simulink model "Thrust_Direction_quad"  (R2013a)
settings: Solver=ode3  StartTime=0.0  StopTime=10.0  FixedStep=t_s  RelTol=1e-3
libraries: quad_lib x2
settings Model: Creator=diogo  LastModifiedBy=diogo

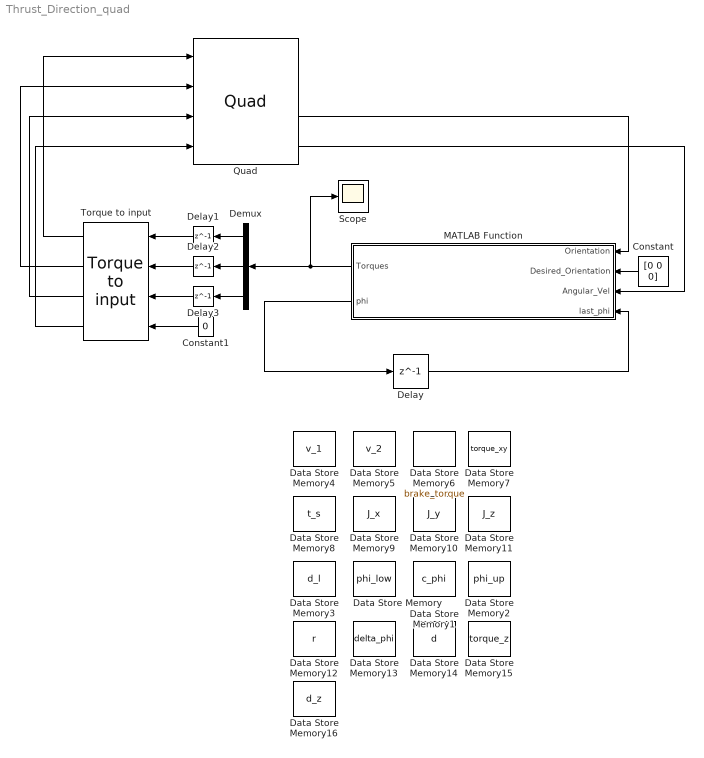
== system Thrust_Direction_quad ==
  Constant : Constant  Value=[0 0 0]
  Constant1 : Constant  Value=0
  Data Store Memory : DataStoreMemory  DataStoreName=phi_low  ReadBeforeWriteMsg=warning  WriteAfterWriteMsg=warning  WriteAfterReadMsg=warning  InitialValue=phi_low  OutDataTypeStr=double
  Data Store Memory1 : DataStoreMemory  DataStoreName=c_phi  ReadBeforeWriteMsg=warning  WriteAfterWriteMsg=warning  WriteAfterReadMsg=warning  InitialValue=c_phi  OutDataTypeStr=double
  Data Store Memory10 : DataStoreMemory  DataStoreName=J_y  ReadBeforeWriteMsg=warning  WriteAfterWriteMsg=warning  WriteAfterReadMsg=warning  InitialValue=J_y  OutDataTypeStr=double
  Data Store Memory11 : DataStoreMemory  DataStoreName=J_z  ReadBeforeWriteMsg=warning  WriteAfterWriteMsg=warning  WriteAfterReadMsg=warning  InitialValue=torque_xy  OutDataTypeStr=double
  Data Store Memory12 : DataStoreMemory  DataStoreName=r  ReadBeforeWriteMsg=warning  WriteAfterWriteMsg=warning  WriteAfterReadMsg=warning  InitialValue=r  OutDataTypeStr=double
  Data Store Memory13 : DataStoreMemory  DataStoreName=delta_phi  ReadBeforeWriteMsg=warning  WriteAfterWriteMsg=warning  WriteAfterReadMsg=warning  InitialValue=delta_phi  OutDataTypeStr=double
  Data Store Memory14 : DataStoreMemory  DataStoreName=d  ReadBeforeWriteMsg=warning  WriteAfterWriteMsg=warning  WriteAfterReadMsg=warning  InitialValue=d  OutDataTypeStr=double
  Data Store Memory15 : DataStoreMemory  DataStoreName=torque_z  ReadBeforeWriteMsg=warning  WriteAfterWriteMsg=warning  WriteAfterReadMsg=warning  InitialValue=torque_z  OutDataTypeStr=double
  Data Store Memory16 : DataStoreMemory  DataStoreName=d_z  ReadBeforeWriteMsg=warning  WriteAfterWriteMsg=warning  WriteAfterReadMsg=warning  InitialValue=d_z  OutDataTypeStr=double
  Data Store Memory2 : DataStoreMemory  DataStoreName=phi_up  ReadBeforeWriteMsg=warning  WriteAfterWriteMsg=warning  WriteAfterReadMsg=warning  InitialValue=phi_up  OutDataTypeStr=double
  Data Store Memory3 : DataStoreMemory  DataStoreName=d_l  ReadBeforeWriteMsg=warning  WriteAfterWriteMsg=warning  WriteAfterReadMsg=warning  InitialValue=d_l  OutDataTypeStr=double
  Data Store Memory4 : DataStoreMemory  DataStoreName=v_1  ReadBeforeWriteMsg=warning  WriteAfterWriteMsg=warning  WriteAfterReadMsg=warning  InitialValue=v_1  OutDataTypeStr=double
  Data Store Memory5 : DataStoreMemory  DataStoreName=v_2  ReadBeforeWriteMsg=warning  WriteAfterWriteMsg=warning  WriteAfterReadMsg=warning  InitialValue=v_2  OutDataTypeStr=double
  Data Store Memory6 : DataStoreMemory  DataStoreName=brake_torque  ReadBeforeWriteMsg=warning  WriteAfterWriteMsg=warning  WriteAfterReadMsg=warning  InitialValue=brake_torque  OutDataTypeStr=double
  Data Store Memory7 : DataStoreMemory  DataStoreName=torque_xy  ReadBeforeWriteMsg=warning  WriteAfterWriteMsg=warning  WriteAfterReadMsg=warning  InitialValue=torque_xy  OutDataTypeStr=double
  Data Store Memory8 : DataStoreMemory  DataStoreName=t_s  ReadBeforeWriteMsg=warning  WriteAfterWriteMsg=warning  WriteAfterReadMsg=warning  InitialValue=t_s  OutDataTypeStr=double
  Data Store Memory9 : DataStoreMemory  DataStoreName=J_x  ReadBeforeWriteMsg=warning  WriteAfterWriteMsg=warning  WriteAfterReadMsg=warning  InitialValue=J_x  OutDataTypeStr=double
  Delay{,1..3} (4 alike) : Delay  DelayLength=1  InitialCondition=0
  Demux : Demux  Outputs=3
  MATLAB Function : MATLAB Function  TreatAsAtomicUnit=on
  Quad : quad_lib/Quad
  Scope : Scope
      settings: YMin=0  YMax=0.11
  Torque to input : quad_lib/PID_quad/Torque to input
  wires:
  Demux/1 -> Delay1/1
  Demux/2 -> Delay2/1
  Demux/3 -> Delay3/1
  Torque to input/4 -> Quad/4
  Torque to input/3 -> Quad/3
  Torque to input/2 -> Quad/2
  Torque to input/1 -> Quad/1
  Constant1/1 -> Torque to input/4
  MATLAB Function/2(phi) -> Delay/1
  Constant/1 -> MATLAB Function/2(Desired_Orientation)
  Delay/1 -> MATLAB Function/4(last_phi)
  MATLAB Function/1(Torques) -> Demux/1, Scope/1
  Delay1/1 -> Torque to input/1
  Delay2/1 -> Torque to input/2
  Delay3/1 -> Torque to input/3
  Quad/3 -> MATLAB Function/1(Orientation)
  Quad/4 -> MATLAB Function/3(Angular_Vel)

== matlab function Thrust_Direction_quad/MATLAB Function ==
  data: Orientation input; Torques output; Desired_Orientation input; Angular_Vel input; last_phi input; phi output; phi_low data_store_memory; c_phi data_store_memory; phi_up data_store_memory; d_l data_store_memory; v_1 data_store_memory; v_2 data_store_memory; brake_torque data_store_memory; torque_xy data_store_memory; t_s data_store_memory; J_x data_store_memory; J_y data_store_memory; J_z data_store_memory; r data_store_memory; delta_phi data_store_memory; d data_store_memory; torque_z data_store_memory; d_z data_store_memory
function [Torques, phi] = Sat_Thrust_Control(Orientation, Desired_Orientation, Angular_Vel, last_phi)
% Computes the command torques that regulates the attitude of a quadrotor
% using the 'Fast and Saturating Thrust Direction Control' method

global phi_low;
global c_phi;
global phi_up;
global d_l;
global v_2;
global v_1;
global brake_torque;
global torque_xy;
global torque_z;
global J_x;
global J_y;
global J_z;
global t_s;
global r;
global delta_phi;
global d;
global d_z;

q = angle_to_quat(Orientation);
q_d = angle_to_quat(Desired_Orientation);

q_e = quat_mult(quat_conjugate(q),q_d);

q_e = q_e.*sign_l(q_e(4));

q_z = get_z_from_quat(q_e);

q_xy = quat_inv_multiply(q,q_z);


phi = 2*acos(q_xy(4));
w_x = Angular_Vel(1);
w_y = Angular_Vel(2);
w_z = Angular_Vel(3);

% Compute the torque field resulting from the potential energy

Torque_phi = 0;

if phi >= 0 && phi <= phi_low
    
    Torque_phi = c_phi * phi;
    
else if phi > phi_low && phi <= phi_up
        
        Torque_phi = c_phi * phi_low;
        
    else if phi > phi_up && phi <= pi
            
            Torque_phi = c_phi*phi_low * (pi-phi)/(pi-phi_up);
            
        end
    end
end


if phi ~= 0
    Torque_field = Torque_phi*(1/(sqrt(1-q_xy(4)^2))); % T(q)
    Torque_field = Torque_field.*[q_xy(1) q_xy(2) 0];
else
    Torque_field = [0 0 0];
end

% % Compute the Damping Injection
% Beta = 0;
% 
% if phi >= 0 && phi <=phi_up
%     Beta = 1;
% else if phi > phi_up && phi <=pi
%         Beta = (pi-phi)/(pi-phi_up);
%     end
% end
% 
% d_xy_low = d_l; % Close to the equilibrium, we add positive damping on all the components of the angular acceleration (to prevent overshooting?)
% 
% 
% % Farther away from the equilibrium, the damping strategy consists in
% % supporting the acceleration while the system is far away from the
% % equilibrium and switching to positive damping when entering the
% % deceleration phase. The switching moment if given by a switch curve that
% % I do not fully understand at the time.
% 
% 
% switch_curve = -sqrt(v_2^2-2*(brake_torque*(phi_low-phi))/J_x);
% 
% phi_dot=(phi-last_phi)*t_s;
% 
% % The acceleration-supporting damping will be positive if the derivative of
% % phi is positive 
% 
% if phi_dot > v_1
%     
%     d_acc = -c_phi*phi_low/phi_dot + brake_torque/phi_dot;
% 
% else if phi_dot > 0 && phi_dot <=v_1
%         
%         d_acc = -c_phi*phi_low/v_1 + brake_torque/v_1; %% to account for a bounded damping
%         
%     else
%         
%         d_acc = 0; %% If the angular speed of phi is negative, the system is moving towards the desired orientation and no damping is required
%         
%     end
% end
% 
% d_dec = -c_phi*phi_low/phi_dot - brake_torque/phi_dot;
% 
% d_mix = d_acc +(phi_dot-r*switch_curve)/((1-r)*switch_curve)*(d_dec-d_acc);
% 
% d_xy=0;
% d_xy_up=0;
% 
% if phi_dot > r*switch_curve
%     
%     d_xy_up = d_acc;
%     
% else if r*switch_curve >= phi_dot && phi_dot > switch_curve
%         
%         d_xy_up = d_mix;
%         
%     else if switch_curve >= phi_dot
%             
%             d_xy_up = d_dec;
%             
%         end
%         
%     end
%     
% end
% 
% % Overal damping obtained by interpolation
% 
% if phi < phi_low
%     
%     d_xy=d_xy_low;
%     
% else if phi >= phi_low && phi < phi_low + delta_phi
%         
%         d_xy = d_xy_low+(phi-phi_low)/delta_phi*(d_xy_up-d_xy_low);
%         
%     else if phi >= phi_low + delta_phi
%             
%             d_xy = d_xy_up;
%             
%         end 
%        
%     end
%     
% end
% 
% 
% % Definition of the Damping matrix
% 
% D_xy = Beta/(1-q_xy(4)^2)*(d_xy*[q_xy(1)^2 q_xy(1)*q_xy(2); q_xy(1)*q_xy(2) q_xy(2)^2] + d*[q_xy(2)^2 -q_xy(1)*q_xy(2); -q_xy(1)*q_xy(2) q_xy(1)^2]);
% 
% % k_1 is the minimum between 1 and the solving of a quadratic equation. If
% % it is less than 1, the control torque in xy is saturated.
% 
% T_x = Torque_field(1);
% T_y = Torque_field(2);
% 
% a = D_xy(1,1)*w_x+D_xy(1,2)*w_y;
% b = D_xy(2,1)*w_x+D_xy(2,2)*w_y;
% 
% if (2*(T_x*a+T_y*b))^2-4*(a^2+b^2)*(T_x^2+T_y^2+torque_xy^2) >= 0
%     k1_a = (2*(T_x*a+T_y*b) - sqrt((2*(T_x*a+T_y*b))^2-4*(a^2+b^2)*(T_x^2+T_y^2+torque_xy^2)))/(2*a^2+b^2);
%     k1_b = (2*(T_x*a+T_y*b) + sqrt((2*(T_x*a+T_y*b))^2-4*(a^2+b^2)*(T_x^2+T_y^2+torque_xy^2)))/(2*a^2+b^2);
%     
%     if k1_a > 0
%         k1 = k1_a;
%     else if k1_b > 0
%             k1 = k1_b;
%         else
%             k1 = 0;
%         end
%     end
% else
%     k1 = 1;
%     
% end
% 
% if k1 > 1
%     k1 = 1;
% end
% 
% k2 = torque_z/abs(d_z*w_z);
% 
% if k2 > 1
%     k2 = 1;
% end
% 
% D = [k1*D_xy zeros(2,1); zeros(1,2) k2*d_z];
% 
% Torques = Torque_field' - D*[w_x;w_y;w_z];
Torques = Torque_field';
